simulink model "Smart_EV_Charging_Station_Project_Simulation"  (R2024b)
settings: Solver=ode23tb  StartTime=0.0  StopTime=4  RelTol=1e-12
undefined symbols (not defined in the file): Ion, Lithium
libraries: spsSeriesRLCBranchLib x34, spsPWMGeneratorDCDCLib x12, spsIdealSwitchLib x12, slpidlib x11, spsGroundLib x10, spsMosfetLib x10, spsIGBTDiodeLib x8, spsDiodeLib x7, spsVoltageMeasurementLib x7, spsBatteryLib x6, spsIGBTLib x6, spsThyristorLib x6
(part 3 of 3)

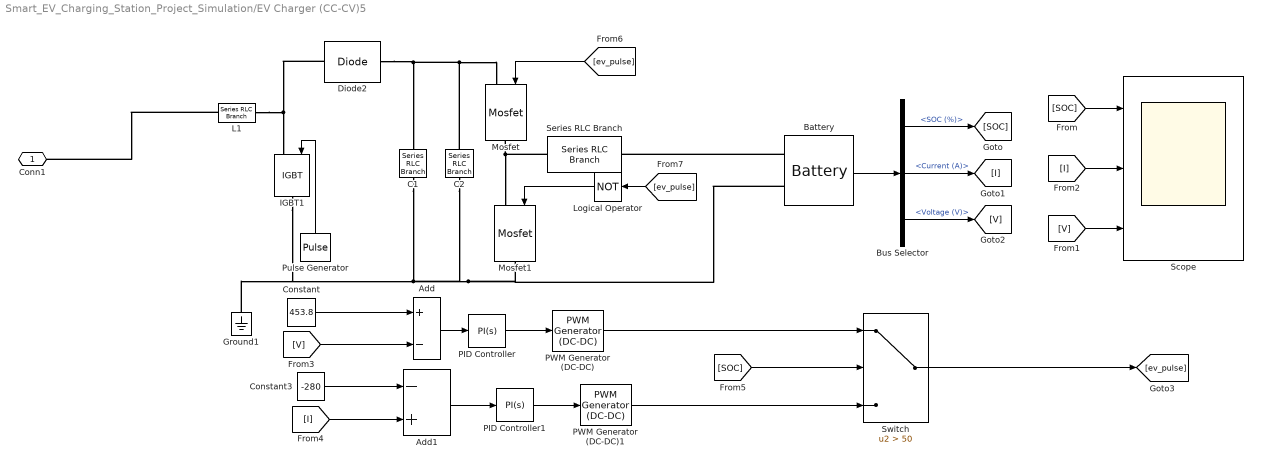
== system Smart_EV_Charging_Station_Project_Simulation/EV Charger (CC-CV)5 ==
  Add : Sum  Inputs=+-
  Add1 : Sum  Inputs=-+
  Battery : spsBatteryLib/Battery  BatType=Lithium-Ion  NomV=400  NomQ=375  SOC=48.25  Batt_Tr=1  PresetModel=on  MaxQ=375  MinV=300  FullV=465.5949  Dis_rate=163.0435  R=0.010667  Normal_OP=339.1304  expZone="[432.1543      18.42391]"
  Bus Selector : BusSelector  OutputSignals=SOC (%),Current (A),Voltage (V)
  C1 : spsSeriesRLCBranchLib/Series RLC Branch  LConnTagsString=__new0  RConnTagsString=__new0  BranchType=C  Resistance=1.0  Inductance=1.0  SetiL0=off  InitialCurrent=0  Capacitance=0.15  Setx0=off  InitialVoltage=0  Measurements=None
  C2 : spsSeriesRLCBranchLib/Series RLC Branch  LConnTagsString=__new0  RConnTagsString=__new0  BranchType=R  Resistance=0.048  Inductance=1.0  SetiL0=off  InitialCurrent=0  Capacitance=100e-6  Setx0=off  InitialVoltage=0  Measurements=Branch voltage
  Constant : Constant  Value=453.8
  Constant3 : Constant  Value=-280
  Diode2 : spsDiodeLib/Diode  Ron=0.001  Lon=0  Vf=0.8  IC=0  UseSnubber=0  Rs=500  Cs=250e-9  Measurements=off
  Ground1 : spsGroundLib/Ground  LConnTagsString=a
  IGBT1 : spsIGBTLib/IGBT  Ron=0.001  Lon=0  Vf=0  Tf=0  Tt=0  IC=0  Rs=1e5  Cs=inf  Measurements=off
  L1 : spsSeriesRLCBranchLib/Series RLC Branch  LConnTagsString=__new0  RConnTagsString=__new0  BranchType=L  Resistance=0.005  Inductance=7e-05  SetiL0=off  InitialCurrent=0  Capacitance=1e-6  Setx0=off  InitialVoltage=0  Measurements=None
  Logical Operator : Logic  Operator=NOT  AllPortsSameDT=off  OutDataTypeStr=boolean
  Mosfet : spsMosfetLib/Mosfet  Ron=0.1  Lon=0  Rd=0.01  Vfd=0  IC=0  Rs=1e5  Cs=inf  Measurements=off
  Mosfet1 : spsMosfetLib/Mosfet  Ron=0.1  Lon=0  Rd=0.01  Vfd=0  IC=0  Rs=1e5  Cs=inf  Measurements=off
  PID Controller : slpidlib/PID Controller  Controller=PI  Form=Parallel  TimeDomain=Continuous-time  UseExternalTs=off  SampleTime=-1  IntegratorMethod=Forward Euler  FilterMethod=Forward Euler  ControllerParametersSource=internal  P=10  I=200  UseKiTs=off  D=0  UseExternalDerivativeSource=off  N=100  UseFilter=on  TunerSelectOption=Transfer Function Based (PID Tuner App)  InitialConditionSource=internal  InitialConditionForIntegrator=0  InitialConditionForFilter=0  DifferentiatorICPrevScaledInput=0  ExternalReset=none  TrackingMode=off  Kt=1  LimitOutput=off  SatLimitsSource=internal  UpperSaturationLimit=inf  LowerSaturationLimit=-inf  LinearizeAsGain=on  AntiWindupMode=none  Kb=1  LimitIntegrator=off  UpperIntegratorSaturationLimit=inf  LowerIntegratorSaturationLimit=-inf  POutMin=[]  POutMax=[]  IOutMin=[]  IOutMax=[]  DOutMin=[]  DOutMax=[]  NOutMin=[]  NOutMax=[]  SumOutMin=[]  SumOutMax=[]  SaturationOutMin=[]  SaturationOutMax=[]  PParamMin=[]  PParamMax=[]  IParamMin=[]  IParamMax=[]  DParamMin=[]  DParamMax=[]  NParamMin=[]  NParamMax=[]  KbParamMin=[]  KbParamMax=[]  KtParamMin=[]  KtParamMax=[]  KbOutMin=[]  KbOutMax=[]  KtOutMin=[]  KtOutMax=[]  IntegratorOutMin=[]  IntegratorOutMax=[]  FilterOutMin=[]  FilterOutMax=[]  SumI1OutMin=[]  SumI1OutMax=[]  SumI2OutMin=[]  SumI2OutMax=[]  SumI3OutMin=[]  SumI3OutMax=[]  SumI4OutMin=[]  SumI4OutMax=[]  SumDOutMin=[]  SumDOutMax=[]  DifferentiatorOutMin=[]  DifferentiatorOutMax=[]  FilterDiffOutCoefMin=[]  FilterDiffOutCoefMax=[]  ReciprocalOutMin=[]  ReciprocalOutMax=[]  SumDenOutMin=[]  SumDenOutMax=[]  SumNumOutMin=[]  SumNumOutMax=[]  DivideOutMin=[]  DivideOutMax=[]  UdiffTsProdOutMin=[]  UdiffTsProdOutMax=[]  NTsProdOutMin=[]  NTsProdOutMax=[]  UintegralTsProdOutMin=[]  UintegralTsProdOutMax=[]  UngainTsProdOutMin=[]  UngainTsProdOutMax=[]  ClampingZeroOutDataTypeStr=Inherit: Inherit via back propagation  ClampingZeroOutMin=[]  ClampingZeroOutMax=[]  FilterDenConstantOutDataTypeStr=Inherit: Inherit via back propagation  FilterDenConstantOutMin=[]  FilterDenConstantOutMax=[]  PCopyOutDataTypeStr=Inherit: Inherit via back propagation  PCopyOutMin=[]  PCopyOutMax=[]  NCopyOutDataTypeStr=Inherit: Inherit via back propagation  NCopyOutMin=[]  NCopyOutMax=[]  IntegratorContinuousStateAttributes=''  IntegratorStateMustResolveToSignalObject=off  IntegratorRTWStateStorageClass=Auto  FilterContinuousStateAttributes=''  FilterStateMustResolveToSignalObject=off  FilterRTWStateStorageClass=Auto  ParallelPVariant=InternalParameters  IdealPVariant=Disabled  IVariant=InternalParameters  DVariant=Disabled  IntegratorVariant=Continuous  SatVariant=Disabled  AWVariant=Passthrough  PCopyVariant=Disabled  TRVariant=Disabled  FdbkBlocksVariant=Forward  IdealPFdbkVariant=Disabled  SatFdbkVariant=Disabled  DerivativeFilterVariant=Disabled  NVariant=Disabled  NCopyVariant=Disabled_SignalSpec  FilterICVariant=Disabled  IntegratorICVariant=InternalICs  ExternalResetVariant=Disabled  TRSumVariant=Passthrough  SumFdbkVariant=Disabled  SumVariant=Sum_PI  TsampFilterVariant=InternalTs  TsampNgainVariant=Passthrough  TsampIntegralVariant=Disabled_SignalSpec  ExternalSaturationOutDataTypeStr=Inherit: Same as second input  DerivativeSourceVariant=Disabled  PreIntVariant=InternalPreInt
  PID Controller1 : slpidlib/PID Controller  Controller=PI  Form=Parallel  TimeDomain=Continuous-time  UseExternalTs=off  SampleTime=-1  IntegratorMethod=Forward Euler  FilterMethod=Forward Euler  ControllerParametersSource=internal  P=0.01  I=2  UseKiTs=off  D=0  UseExternalDerivativeSource=off  N=100  UseFilter=on  TunerSelectOption=Transfer Function Based (PID Tuner App)  InitialConditionSource=internal  InitialConditionForIntegrator=0  InitialConditionForFilter=0  DifferentiatorICPrevScaledInput=0  ExternalReset=none  TrackingMode=off  Kt=1  LimitOutput=off  SatLimitsSource=internal  UpperSaturationLimit=inf  LowerSaturationLimit=-inf  LinearizeAsGain=on  AntiWindupMode=none  Kb=1  LimitIntegrator=off  UpperIntegratorSaturationLimit=inf  LowerIntegratorSaturationLimit=-inf  POutMin=[]  POutMax=[]  IOutMin=[]  IOutMax=[]  DOutMin=[]  DOutMax=[]  NOutMin=[]  NOutMax=[]  SumOutMin=[]  SumOutMax=[]  SaturationOutMin=[]  SaturationOutMax=[]  PParamMin=[]  PParamMax=[]  IParamMin=[]  IParamMax=[]  DParamMin=[]  DParamMax=[]  NParamMin=[]  NParamMax=[]  KbParamMin=[]  KbParamMax=[]  KtParamMin=[]  KtParamMax=[]  KbOutMin=[]  KbOutMax=[]  KtOutMin=[]  KtOutMax=[]  IntegratorOutMin=[]  IntegratorOutMax=[]  FilterOutMin=[]  FilterOutMax=[]  SumI1OutMin=[]  SumI1OutMax=[]  SumI2OutMin=[]  SumI2OutMax=[]  SumI3OutMin=[]  SumI3OutMax=[]  SumI4OutMin=[]  SumI4OutMax=[]  SumDOutMin=[]  SumDOutMax=[]  DifferentiatorOutMin=[]  DifferentiatorOutMax=[]  FilterDiffOutCoefMin=[]  FilterDiffOutCoefMax=[]  ReciprocalOutMin=[]  ReciprocalOutMax=[]  SumDenOutMin=[]  SumDenOutMax=[]  SumNumOutMin=[]  SumNumOutMax=[]  DivideOutMin=[]  DivideOutMax=[]  UdiffTsProdOutMin=[]  UdiffTsProdOutMax=[]  NTsProdOutMin=[]  NTsProdOutMax=[]  UintegralTsProdOutMin=[]  UintegralTsProdOutMax=[]  UngainTsProdOutMin=[]  UngainTsProdOutMax=[]  ClampingZeroOutDataTypeStr=Inherit: Inherit via back propagation  ClampingZeroOutMin=[]  ClampingZeroOutMax=[]  FilterDenConstantOutDataTypeStr=Inherit: Inherit via back propagation  FilterDenConstantOutMin=[]  FilterDenConstantOutMax=[]  PCopyOutDataTypeStr=Inherit: Inherit via back propagation  PCopyOutMin=[]  PCopyOutMax=[]  NCopyOutDataTypeStr=Inherit: Inherit via back propagation  NCopyOutMin=[]  NCopyOutMax=[]  IntegratorContinuousStateAttributes=''  IntegratorStateMustResolveToSignalObject=off  IntegratorRTWStateStorageClass=Auto  FilterContinuousStateAttributes=''  FilterStateMustResolveToSignalObject=off  FilterRTWStateStorageClass=Auto  ParallelPVariant=InternalParameters  IdealPVariant=Disabled  IVariant=InternalParameters  DVariant=Disabled  IntegratorVariant=Continuous  SatVariant=Disabled  AWVariant=Passthrough  PCopyVariant=Disabled  TRVariant=Disabled  FdbkBlocksVariant=Forward  IdealPFdbkVariant=Disabled  SatFdbkVariant=Disabled  DerivativeFilterVariant=Disabled  NVariant=Disabled  NCopyVariant=Disabled_SignalSpec  FilterICVariant=Disabled  IntegratorICVariant=InternalICs  ExternalResetVariant=Disabled  TRSumVariant=Passthrough  SumFdbkVariant=Disabled  SumVariant=Sum_PI  TsampFilterVariant=InternalTs  TsampNgainVariant=Passthrough  TsampIntegralVariant=Disabled_SignalSpec  ExternalSaturationOutDataTypeStr=Inherit: Same as second input  DerivativeSourceVariant=Disabled  PreIntVariant=InternalPreInt
  PWM Generator (DC-DC) : spsPWMGeneratorDCDCLib/PWM Generator (DC-DC)  Fsw=10e3  Ts=20e-6
  PWM Generator (DC-DC)1 : spsPWMGeneratorDCDCLib/PWM Generator (DC-DC)  Fsw=10e3  Ts=20e-6
  Pulse Generator : DiscretePulseGenerator  PulseType=Time based  Period=1/10000  PulseWidth=37
  Scope : Scope  NumInputPorts=3
  Series RLC Branch : spsSeriesRLCBranchLib/Series RLC Branch  LConnTagsString=__new0  RConnTagsString=__new0  BranchType=RL  Resistance=0.05  Inductance=10e-3  SetiL0=off  InitialCurrent=0  Capacitance=1e-6  Setx0=off  InitialVoltage=0  Measurements=None
  Switch : Switch  Criteria=u2 > Threshold  Threshold=50  SaturateOnIntegerOverflow=off  InputSameDT=off
  Conn1 : PMIOPort  Side=Left
  wires:
  PWM Generator (DC-DC)1/1 -> Switch/3
  Constant/1 -> Add/1
  PID Controller/1 -> PWM Generator (DC-DC)/1
  Logical Operator/1 -> Mosfet1/1
  [ev_pulse] -> Mosfet/1
  Switch/1 -> [ev_pulse]
  [V] -> Add/2
  PID Controller1/1 -> PWM Generator (DC-DC)1/1
  Constant3/1 -> Add1/1
  Add/1 -> PID Controller/1
  Bus Selector/1 -> [SOC]  "<SOC (%)>"
  [V] -> Scope/3
  [I] -> Scope/2
  Add1/1 -> PID Controller1/1
  PWM Generator (DC-DC)/1 -> Switch/1
  [I] -> Add1/2
  Battery/1 -> Bus Selector/1
  [SOC] -> Switch/2
  Bus Selector/3 -> [V]  "<Voltage (V)>"
  [SOC] -> Scope/1
  Bus Selector/2 -> [I]  "<Current (A)>"
  Pulse Generator/1 -> IGBT1/1
  [ev_pulse] -> Logical Operator/1
  connections:
  C1/RConn1 -- Ground1/LConn1 -- IGBT1/RConn1 -- C2/RConn1 -- Battery/LConn2 -- Mosfet1/RConn1
  Series RLC Branch/LConn1 -- Mosfet1/LConn1 -- Mosfet/RConn1
  Battery/LConn1 -- Series RLC Branch/RConn1
  L1/LConn1 -- Conn1/RConn1
  L1/RConn1 -- Diode2/LConn1 -- IGBT1/LConn1
  C2/LConn1 -- Diode2/RConn1 -- C1/LConn1 -- Mosfet/LConn1

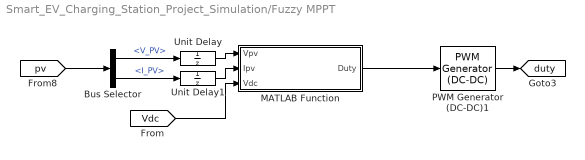
== system Smart_EV_Charging_Station_Project_Simulation/Fuzzy MPPT ==
  Bus Selector : BusSelector  OutputSignals=V_PV,I_PV
  MATLAB Function : MATLAB Function  TreatAsAtomicUnit=on
  PWM Generator (DC-DC)1 : spsPWMGeneratorDCDCLib/PWM Generator (DC-DC)  Fsw=10000  Ts=0
  Unit Delay : UnitDelay  SampleTime=1e-6  HasFrameUpgradeWarning=on
  Unit Delay1 : UnitDelay  SampleTime=1e-6  HasFrameUpgradeWarning=on
  tag scope: duty=global
  wires:
  MATLAB Function/1(Duty) -> PWM Generator (DC-DC)1/1
  Bus Selector/2 -> Unit Delay1/1  "<I_PV>"
  Unit Delay/1 -> MATLAB Function/1(Vpv)
  Bus Selector/1 -> Unit Delay/1  "<V_PV>"
  PWM Generator (DC-DC)1/1 -> [duty]
  [pv] -> Bus Selector/1
  [Vdc] -> MATLAB Function/3(Vdc)
  Unit Delay1/1 -> MATLAB Function/2(Ipv)

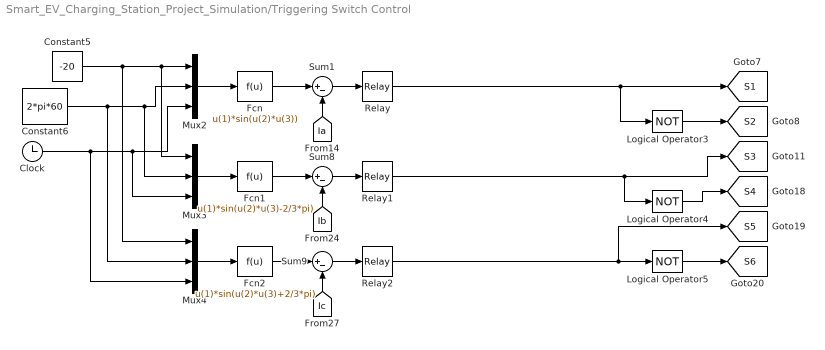
== system Smart_EV_Charging_Station_Project_Simulation/Triggering Switch Control ==
  Clock : Clock
  Constant5 : Constant  Value=-20
  Constant6 : Constant  Value=2*pi*60
  Fcn : Fcn  Expr=u(1)*sin(u(2)*u(3))
  Fcn1 : Fcn  Expr=u(1)*sin(u(2)*u(3)-2/3*pi)
  Fcn2 : Fcn  Expr=u(1)*sin(u(2)*u(3)+2/3*pi)
  Logical Operator3 : Logic  Operator=NOT  AllPortsSameDT=off  OutDataTypeStr=boolean
  Logical Operator4 : Logic  Operator=NOT  AllPortsSameDT=off  OutDataTypeStr=boolean
  Logical Operator5 : Logic  Operator=NOT  AllPortsSameDT=off  OutDataTypeStr=boolean
  Mux2 : Mux  Inputs=3
  Mux3 : Mux  Inputs=3
  Mux4 : Mux  Inputs=3
  Relay : Relay  OnSwitchValue=0.5  OffSwitchValue=-0.5
  Relay1 : Relay  OnSwitchValue=0.5  OffSwitchValue=-0.5
  Relay2 : Relay  OnSwitchValue=0.5  OffSwitchValue=-0.5
  Sum1 : Sum  Inputs=|+-
  Sum8 : Sum  Inputs=|+-
  Sum9 : Sum  Inputs=|+-
  tag scope: S1=global, S2=global, S3=global, S4=global, S5=global, S6=global
  wires:
  Relay/1 -> [S1], Logical Operator3/1
  Logical Operator5/1 -> [S6]
  Sum8/1 -> Relay1/1
  [Ib] -> Sum8/2
  Fcn/1 -> Sum1/1
  Logical Operator4/1 -> [S4]
  Mux2/1 -> Fcn/1
  Sum1/1 -> Relay/1
  Clock/1 -> Mux4/3, Mux3/3, Mux2/3
  [Ia] -> Sum1/2
  Relay2/1 -> [S5], Logical Operator5/1
  Mux4/1 -> Fcn2/1
  [Ic] -> Sum9/2
  Logical Operator3/1 -> [S2]
  Fcn2/1 -> Sum9/1
  Constant5/1 -> Mux4/1, Mux3/1, Mux2/1
  Relay1/1 -> [S3], Logical Operator4/1
  Mux3/1 -> Fcn1/1
  Sum9/1 -> Relay2/1
  Fcn1/1 -> Sum8/1
  Constant6/1 -> Mux4/2, Mux3/2, Mux2/2

== matlab function Smart_EV_Charging_Station_Project_Simulation/MATLAB Function ==
  data: P_pv input; ev_pv_1 output; constant input; Soc input; ev_grid_1 output; ev_pv_2 output; ev_grid_2 output; ev_pv_3 output; ev_grid_3 output; ev_pv_4 output; ev_grid_4 output; ev_pv_5 output; ev_grid_5 output; Micro_grid output
function [ev_pv_1, ev_grid_1, ev_pv_2, ev_grid_2, ev_pv_3, ev_grid_3, ev_pv_4, ev_grid_4, ev_pv_5, ev_grid_5, Micro_grid] = EnergyManagementBlock(P_pv, constant, Soc)
% EnergyManagementBlock assigns EV chargers to either PV or grid and controls a Micro_grid switch.
%
% Inputs:
%   P_pv    - Solar power (in Watts)
%   constant- A value from 0 to 5 indicating active EV chargers.
%   Soc     - Battery State-of-Charge (in percentage)
%
% Outputs:
%   For each EV charger i (1 to 5):
%       ev_pv_i   - 1 if charger i is connected to the PV bus, 0 otherwise.
%       ev_grid_i - 1 if charger i is connected to the grid, 0 otherwise.
%   Micro_grid  - 1 if the Microgrid is switched on, 0 otherwise.
%
% Conditions:
%   1. Initially, Micro_grid is off.
%   2. If constant == 0:
%        - Check the battery SOC.
%        - If SOC is 80% or above, turn on Micro_grid.
%        - All EV charger outputs are off.
%   3. If constant > 0:
%        - Convert P_pv from Watts to kW and add an offset of 30.
%        - Each EV charger is rated at 150 kW.
%        - Assign as many chargers as possible to PV without exceeding available PV power.
%        - The remaining active chargers are fed from the grid.
%        - Micro_grid remains off.

% Initialize EV charger outputs to off (0)
ev_pv   = zeros(1,5);
ev_grid = zeros(1,5);

% Default: Micro_grid is off.
Micro_grid = 0;

if constant == 0
    % No EV chargers active.
    % Check battery SOC: if SOC is 80% or above, turn on Micro_grid.
    if Soc >= 80
        Micro_grid = 1;
    end
    % EV charger outputs remain off.
else
    % EV chargers are active.
    % Convert solar power from W to kW with an additional 50 kW offset.
    P_pv_kW = (P_pv / 1000) + 50;
    
    % Each charger requires 150 kW.
    % Determine how many chargers can be powered by PV.
    maxPVChargers = floor(P_pv_kW / 150);
    
    % Loop through each charger (1 to 5)
    for i = 1:5
        if i <= constant
            % Active charger.
            if i <= maxPVChargers
                % Assign charger to PV bus.
                ev_pv(i) = 1;
                ev_grid(i) = 0;
            else
                % Not enough PV power: assign charger to grid.
                ev_pv(i) = 0;
                ev_grid(i) = 1;
            end
        else
            % Inactive charger: both outputs remain off.
            ev_pv(i) = 0;
            ev_grid(i) = 0;
        end
    end
    % In this mode, Micro_grid remains off.
end

% Introduce a delay of 0.1 seconds (100 milliseconds)
%pause(0.1);

% Map array values to individual output variables
ev_pv_1   = ev_pv(1);
ev_grid_1 = ev_grid(1);
ev_pv_2   = ev_pv(2);
ev_grid_2 = ev_grid(2);
ev_pv_3   = ev_pv(3);
ev_grid_3 = ev_grid(3);
ev_pv_4   = ev_pv(4);
ev_grid_4 = ev_grid(4);
ev_pv_5   = ev_pv(5);
ev_grid_5 = ev_grid(5);

end

== matlab function Smart_EV_Charging_Station_Project_Simulation/Fuzzy MPPT/MATLAB Function ==
  data: Vpv input; Duty output; Ipv input; Vdc input
function Duty = fuzzy_mppt(Vpv, Ipv, Vdc)
    % Persistent Variables to Store Previous Values
    persistent P_prev  E_prev Duty_prev;
    
    % Initialize Persistent Variables on First Run
    if isempty(P_prev)
        P_prev = 0;         % Previous Power
        E_prev = 0;         % Previous Error
        Duty_prev = 0.204;  % Initial Duty Cycle (20.4%)
    end
    
    % Calculate Instantaneous PV Power
    Ppv = Vpv * Ipv;
    
    % Compute Error (Difference in PV Power)
    E = Ppv - P_prev;
    
    % Compute Change in Error (Rate of Change of Power)
    dE = E - E_prev;

    % Define 7-Level Fuzzy Membership Functions for E and dE
    NB = -3; NM = -2; NS = -1; 
    Z = 0; 
    PS = 1; PM = 2; PB = 3;
    
    % Define error thresholds for improved accuracy
    err_thresholds = [-20, -10, -5, 0, 5, 10, 20];  % Fuzzy boundaries
    d_err_thresholds = [-15, -8, -4, 0, 4, 8, 15];  % Change in power boundaries
    
    % Assign fuzzy levels based on error
    if E < err_thresholds(1)
        E_fuzzy = NB;
    elseif E < err_thresholds(2)
        E_fuzzy = NM;
    elseif E < err_thresholds(3)
        E_fuzzy = NS;
    elseif E < err_thresholds(4)
        E_fuzzy = Z;
    elseif E < err_thresholds(5)
        E_fuzzy = PS;
    elseif E < err_thresholds(6)
        E_fuzzy = PM;
    else
        E_fuzzy = PB;
    end
    
    % Assign fuzzy levels based on change in error
    if dE < d_err_thresholds(1)
        dE_fuzzy = NB;
    elseif dE < d_err_thresholds(2)
        dE_fuzzy = NM;
    elseif dE < d_err_thresholds(3)
        dE_fuzzy = NS;
    elseif dE < d_err_thresholds(4)
        dE_fuzzy = Z;
    elseif dE < d_err_thresholds(5)
        dE_fuzzy = PS;
    elseif dE < d_err_thresholds(6)
        dE_fuzzy = PM;
    else
        dE_fuzzy = PB;
    end

    % **Fuzzy Inference System (7x7 Rule Base)**
    % Rule base: Mapping E_fuzzy and dE_fuzzy to dD
    fuzzy_rule_table = [  NB, NB, NM, NS, Z,  PS, PM;
                          NB, NB, NM, NS, Z,  PS, PM;
                          NM, NM, NS, Z,  PS, PM, PB;
                          NS, NS, Z,  Z,  Z,  PS, PS;
                          Z,  Z,  PS, Z,  Z,  NS, NS;
                          PS, PM, PB, PS, Z,  NM, NM;
                          PM, PB, PB, PM, Z,  NB, NB  ];

    % Get dD from fuzzy rule table
    dD = fuzzy_rule_table(E_fuzzy + 4, dE_fuzzy + 4); % Offset by 4 to index correctly

    % **Adaptive Scaling Factor for Duty Cycle Change**
    base_scaling = 0.0004;  % Smaller step changes for ultra-fine control
    
    % Adaptive Scaling: Reduce when power changes are high
    if abs(dE) > 10
        scaling_factor = base_scaling * 0.5;  % Reduce step size when fluctuations are high
    else
        scaling_factor = base_scaling;  % Normal operation
    end
    
    dD_actual = dD * scaling_factor;

    % **Boost Converter Output Voltage Stability Control**
    Vdc_ref = 405;  % Target Boost Output Voltage
    Vdc_tolerance = 1;  % Allowable voltage range (strict but controlled)

    % **Create a "Dead Zone" Around 400V**
    % This prevents unnecessary tiny duty cycle changes due to noise
    if abs(Vdc - Vdc_ref) < 1  
        dD_actual = 0;  % Hold duty cycle constant in the "safe zone"
    elseif Vdc > Vdc_ref + Vdc_tolerance   % If Vdc is too high, slightly decrease duty cycle
        dD_actual = dD_actual - 0.00005;  % Very fine correction
    elseif Vdc < Vdc_ref - Vdc_tolerance   % If Vdc is too low, slightly increase duty cycle
        dD_actual = dD_actual + 0.00005;  % Very fine correction
    end
    
    % **Update Duty Cycle with Clamping**
    Duty = Duty_prev + dD_actual;

    % **Clamp Duty Cycle Between Safe Limits (Preventing Instability)**
    if Duty > 0.85   % Reduce max limit to prevent excessive boost voltage
        Duty = 0.85;
    elseif Duty < 0.15   % Ensure enough switching action
        Duty = 0.15;
    end

    % **Store Updated Values for Next Iteration**
    P_prev = Ppv;
    E_prev = E;
    Duty_prev = Duty; % Store Updated Duty Cycle
end
